simulink model "InnerController"  (R2016b)
settings: Solver=FixedStepAuto  StartTime=0.0  StopTime=t  FixedStep=Ts  RelTol=1e-3
model workspace (MAT data in the model file):
  index = Simulink.Signal
  index.DataType = 'double'
  index.Dimensions = 1
  index.DimensionsMode = 'Fixed'
  index.Complexity = 'real'
  index.SampleTime = -1
  index.SamplingMode = 'auto'
  index.InitialValue = '1'
values from neighbouring files (symbols this model uses):
  dx = 2.86    [Parameters.m]    (also in PlotControllersPerformance.m = dx_rand(i))
  dy = 32.5    [Parameters.m]    (also in PlotControllersPerformance.m = dy_rand(i))
  dyaw = 0.26285    [Parameters.m]    (also in PlotControllersPerformance.m = dyaw_rand(i))
  enable_disturbance = 1    [PlotControllersPerformance.m]
  F_lqr = Fe_lqr(1:2,1:3)    [ControllersDesign.m]
  F_rob = -info.KFI(1:2,1:3)    [ControllersDesign.m]
  FI_lqr = Fe_lqr(1:2,4:5)    [ControllersDesign.m]
  FI_rob = -info.KFI(1:2,4:5)    [ControllersDesign.m]
  Iz = 1.10675    [Parameters.m]    (also in PlotControllersPerformance.m = Iz_rand(i))
  l1 = 0.05    [Parameters.m]    (also in PlotControllersPerformance.m = l1_rand(i))
  l2 = 0.05    [Parameters.m]    (also in PlotControllersPerformance.m = l2_rand(i))
  m = 13    [Parameters.m]    (also in PlotControllersPerformance.m = m_rand(i))
  noise_power_xbdot = 0.000001    (= 1e-06)    [PlotControllersPerformance.m]
  noise_power_yaw = 0.0000001    (= 1e-07)    [PlotControllersPerformance.m]
  noise_power_yawdot = 0.000001    (= 1e-06)    [PlotControllersPerformance.m]
  refXdot = 1    [PlotControllersPerformance.m]
  refYaw = 1    [PlotControllersPerformance.m]
  sineAmplitude = 0.5    [PlotControllersPerformance.m]
  sineFrequency = sineFrequency_rand(i)    [PlotControllersPerformance.m]
  time_step = 10    [PlotControllersPerformance.m]
  Ts = 0.05    [Parameters.m]
  xbDisturbance = xbDisturbance_rand(i)    [PlotControllersPerformance.m]
  yawDisturbance = yawDisturbance_rand(i)    [PlotControllersPerformance.m]
undefined symbols (not defined in the file or in its folder): DiscIntNeverNeededParam
libraries: simulink x6
settings Model: Creator=USUARIO  LastModifiedBy=USUARIO
settings DataIOCC: Refine=100

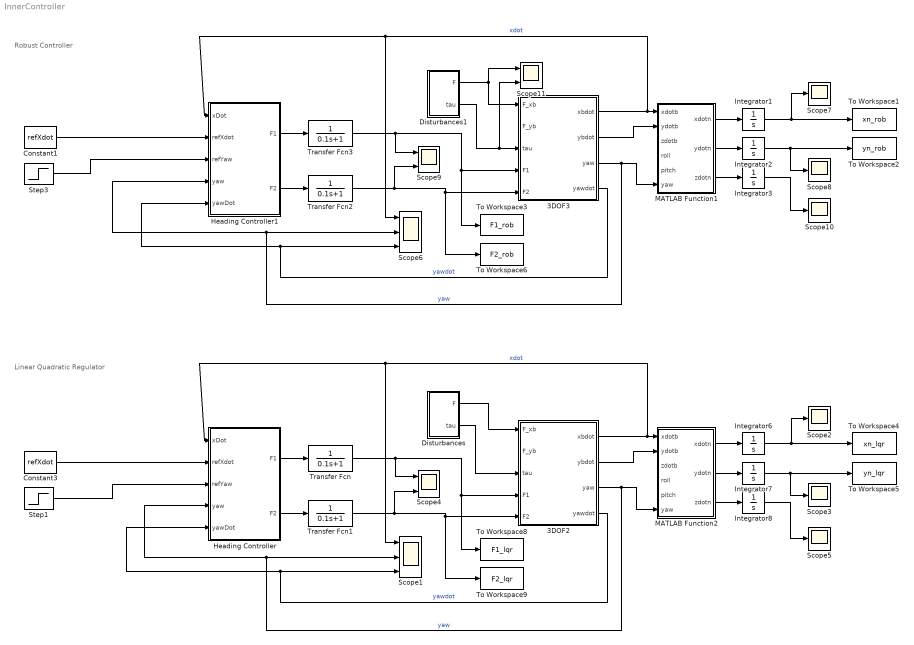
== system InnerController ==
  note: Linear Quadratic Regulator
  note: Robust Controller
  3DOF2 : Subsystem
  3DOF3 : Subsystem
  Constant1 : Constant  Value=refXdot
  Constant3 : Constant  Value=refXdot
  Disturbances : Subsystem
  Disturbances1 : Subsystem
  Heading Controller : Subsystem
  Heading Controller1 : Subsystem
  Integrator{1..3,6..8} (6 alike) : Integrator
  MATLAB Function1 : MATLAB Function  TreatAsAtomicUnit=on
  MATLAB Function2 : MATLAB Function  TreatAsAtomicUnit=on
  Scope1 : Scope  NumInputPorts=3
  Scope{2..3,5,7..8,10} (6 alike) : Scope
  Scope11 : Scope  NumInputPorts=2
  Scope4 : Scope  NumInputPorts=2
  Scope6 : Scope  NumInputPorts=3
  Scope9 : Scope  NumInputPorts=2
  Step1 : Step  Time=time_step  After=refYaw  SampleTime=0
  Step3 : Step  Time=time_step  After=refYaw  SampleTime=0
  To Workspace1 : ToWorkspace  VariableName=xn_rob  SaveFormat=Timeseries  SampleTime=-1
  To Workspace2 : ToWorkspace  VariableName=yn_rob  SaveFormat=Timeseries  SampleTime=-1
  To Workspace3 : ToWorkspace  VariableName=F1_rob  SaveFormat=Timeseries  SampleTime=Ts
  To Workspace4 : ToWorkspace  VariableName=xn_lqr  SaveFormat=Timeseries  SampleTime=-1
  To Workspace5 : ToWorkspace  VariableName=yn_lqr  SaveFormat=Timeseries  SampleTime=-1
  To Workspace6 : ToWorkspace  VariableName=F2_rob  SaveFormat=Timeseries  SampleTime=Ts
  To Workspace8 : ToWorkspace  VariableName=F1_lqr  SaveFormat=Timeseries  SampleTime=-1
  To Workspace9 : ToWorkspace  VariableName=F2_lqr  SaveFormat=Timeseries  SampleTime=-1
  Transfer Fcn{,1..3} (4 alike) : TransferFcn  Denominator=[0.1 1]
  wires:
  3DOF2/1(xbdot) -> Scope1/1, Heading Controller/1(xDot), MATLAB Function2/1(xdotb)  "xdot"
  3DOF2/2(ybdot) -> MATLAB Function2/2(ydotb)
  3DOF2/3(yaw) -> MATLAB Function2/6(yaw), Scope1/2, Heading Controller/4(yaw)  "yaw"
  Integrator6/1 -> Scope2/1, To Workspace4/1
  Integrator7/1 -> Scope3/1, To Workspace5/1
  MATLAB Function2/3(zdotn) -> Integrator8/1
  3DOF2/4(yawdot) -> Heading Controller/5(yawDot), Scope1/3  "yawdot"
  Heading Controller/2(F2) -> Transfer Fcn1/1
  Heading Controller/1(F1) -> Transfer Fcn/1
  MATLAB Function2/1(xdotn) -> Integrator6/1
  MATLAB Function2/2(ydotn) -> Integrator7/1
  Integrator8/1 -> Scope5/1
  Constant3/1 -> Heading Controller/2(refXdot)
  Step1/1 -> Heading Controller/3(refYaw)
  3DOF3/1(xbdot) -> MATLAB Function1/1(xdotb), Scope6/1, Heading Controller1/1(xDot)  "xdot"
  3DOF3/2(ybdot) -> MATLAB Function1/2(ydotb)
  3DOF3/3(yaw) -> Scope6/2, Heading Controller1/4(yaw), MATLAB Function1/6(yaw)  "yaw"
  Integrator1/1 -> To Workspace1/1, Scope7/1
  Integrator2/1 -> To Workspace2/1, Scope8/1
  MATLAB Function1/3(zdotn) -> Integrator3/1
  3DOF3/4(yawdot) -> Scope6/3, Heading Controller1/5(yawDot)  "yawdot"
  Heading Controller1/2(F2) -> Transfer Fcn2/1
  Heading Controller1/1(F1) -> Transfer Fcn3/1
  MATLAB Function1/1(xdotn) -> Integrator1/1
  MATLAB Function1/2(ydotn) -> Integrator2/1
  Integrator3/1 -> Scope10/1
  Constant1/1 -> Heading Controller1/2(refXdot)
  Step3/1 -> Heading Controller1/3(refYaw)
  Transfer Fcn/1 -> Scope4/1, 3DOF2/4(F1), To Workspace8/1
  Transfer Fcn1/1 -> Scope4/2, 3DOF2/5(F2), To Workspace9/1
  Transfer Fcn2/1 -> 3DOF3/5(F2), To Workspace6/1, Scope9/2
  Transfer Fcn3/1 -> 3DOF3/4(F1), To Workspace3/1, Scope9/1
  Disturbances1/1(F) -> 3DOF3/1(F_xb), Scope11/1
  Disturbances1/2(tau) -> Scope11/2, 3DOF3/3(tau)
  Disturbances/1(F) -> 3DOF2/1(F_xb)
  Disturbances/2(tau) -> 3DOF2/3(tau)

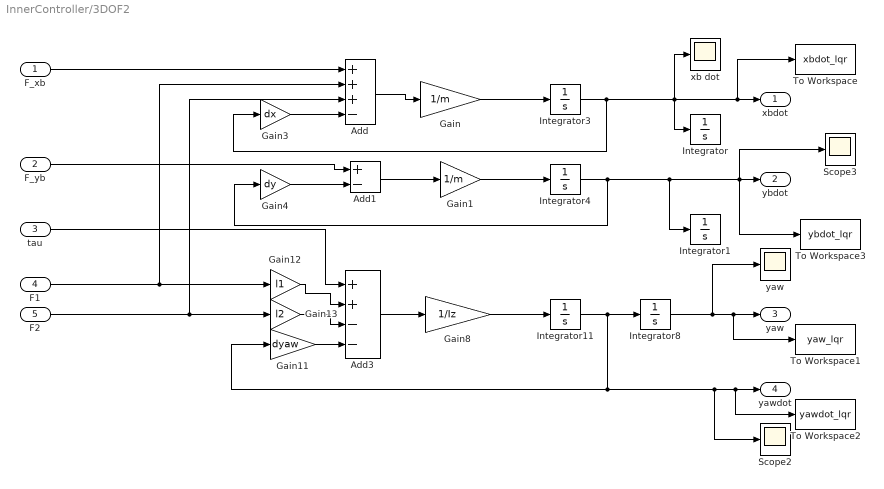
== system InnerController/3DOF2 ==
  F_xb : Inport
  F_yb : Inport  Port=2
  tau : Inport  Port=3
  F1 : Inport  Port=4
  F2 : Inport  Port=5
  Add : Sum  Inputs=+++-
  Add1 : Sum  Inputs=+-
  Add3 : Sum  Inputs=++--
  Gain : Gain  Gain=1/m
  Gain1 : Gain  Gain=1/m
  Gain11 : Gain  Gain=dyaw
  Gain12 : Gain  Gain=l1
  Gain13 : Gain  Gain=l2
  Gain3 : Gain  Gain=dx
  Gain4 : Gain  Gain=dy
  Gain8 : Gain  Gain=1/Iz
  Integrator{,1,3..4,8,11} (6 alike) : Integrator
  Scope2 : Scope
  Scope3 : Scope
  To Workspace : ToWorkspace  VariableName=xbdot_lqr  SaveFormat=Timeseries  SampleTime=Ts
  To Workspace1 : ToWorkspace  VariableName=yaw_lqr  SaveFormat=Timeseries  SampleTime=Ts
  To Workspace2 : ToWorkspace  VariableName=yawdot_lqr  SaveFormat=Timeseries  SampleTime=Ts
  To Workspace3 : ToWorkspace  VariableName=ybdot_lqr  SaveFormat=Timeseries  SampleTime=Ts
  xb dot : Scope
  "yaw " : Scope
  xbdot : Outport
  ybdot : Outport  Port=2
  yaw : Outport  Port=3
  yawdot : Outport  Port=4
  wires:
  Integrator11/1 -> Scope2/1, To Workspace2/1, yawdot/1, Gain11/1, Integrator8/1
  Gain8/1 -> Integrator11/1
  Gain4/1 -> Add1/2
  Gain1/1 -> Integrator4/1
  Gain3/1 -> Add/4
  Add/1 -> Gain/1
  Gain/1 -> Integrator3/1
  Gain12/1 -> Add3/2
  Add3/1 -> Gain8/1
  Gain11/1 -> Add3/4
  Gain13/1 -> Add3/3
  Integrator3/1 -> xb dot/1, Integrator/1, To Workspace/1, xbdot/1, Gain3/1
  Integrator4/1 -> Gain4/1, Integrator1/1, To Workspace3/1, ybdot/1, Scope3/1
  Integrator8/1 -> "yaw "/1, To Workspace1/1, yaw/1
  F1/1 -> Add/2, Gain12/1
  F2/1 -> Add/3, Gain13/1
  Add1/1 -> Gain1/1
  F_yb/1 -> Add1/1
  F_xb/1 -> Add/1
  tau/1 -> Add3/1

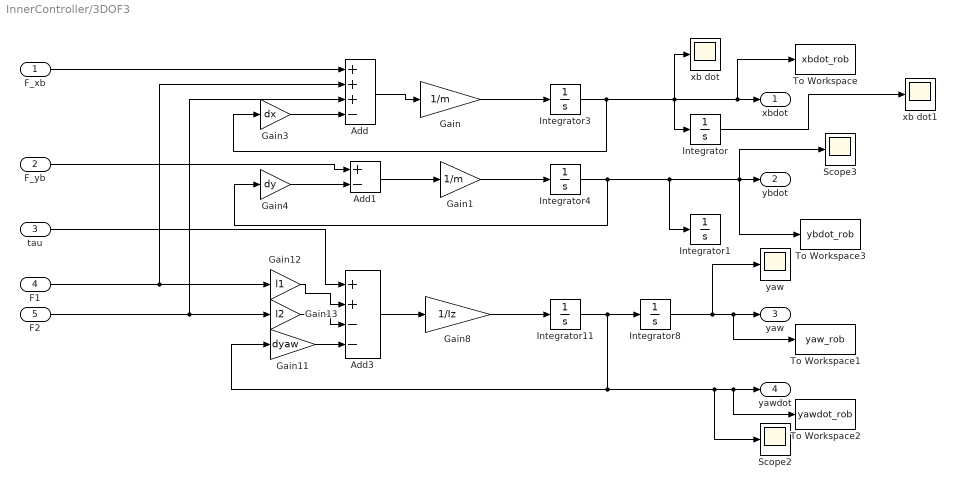
== system InnerController/3DOF3 ==
  F_xb : Inport
  F_yb : Inport  Port=2
  tau : Inport  Port=3
  F1 : Inport  Port=4
  F2 : Inport  Port=5
  Add : Sum  Inputs=+++-
  Add1 : Sum  Inputs=+-
  Add3 : Sum  Inputs=++--
  Gain : Gain  Gain=1/m
  Gain1 : Gain  Gain=1/m
  Gain11 : Gain  Gain=dyaw
  Gain12 : Gain  Gain=l1
  Gain13 : Gain  Gain=l2
  Gain3 : Gain  Gain=dx
  Gain4 : Gain  Gain=dy
  Gain8 : Gain  Gain=1/Iz
  Integrator{,1,3..4,8,11} (6 alike) : Integrator
  Scope2 : Scope
  Scope3 : Scope
  To Workspace : ToWorkspace  VariableName=xbdot_rob  SaveFormat=Timeseries  SampleTime=Ts
  To Workspace1 : ToWorkspace  VariableName=yaw_rob  SaveFormat=Timeseries  SampleTime=Ts
  To Workspace2 : ToWorkspace  VariableName=yawdot_rob  SaveFormat=Timeseries  SampleTime=Ts
  To Workspace3 : ToWorkspace  VariableName=ybdot_rob  SaveFormat=Timeseries  SampleTime=Ts
  xb dot : Scope
  xb dot1 : Scope
  "yaw " : Scope
  xbdot : Outport
  ybdot : Outport  Port=2
  yaw : Outport  Port=3
  yawdot : Outport  Port=4
  wires:
  tau/1 -> Add3/1
  F_xb/1 -> Add/1
  F_yb/1 -> Add1/1
  Add1/1 -> Gain1/1
  F2/1 -> Gain13/1, Add/3
  F1/1 -> Gain12/1, Add/2
  Integrator8/1 -> yaw/1, To Workspace1/1, "yaw "/1
  Integrator4/1 -> Scope3/1, ybdot/1, To Workspace3/1, Integrator1/1, Gain4/1
  Integrator3/1 -> Gain3/1, xbdot/1, To Workspace/1, Integrator/1, xb dot/1
  Gain13/1 -> Add3/3
  Gain11/1 -> Add3/4
  Add3/1 -> Gain8/1
  Gain12/1 -> Add3/2
  Gain/1 -> Integrator3/1
  Add/1 -> Gain/1
  Gain3/1 -> Add/4
  Gain1/1 -> Integrator4/1
  Gain4/1 -> Add1/2
  Gain8/1 -> Integrator11/1
  Integrator11/1 -> Integrator8/1, Gain11/1, To Workspace2/1, yawdot/1, Scope2/1
  Integrator/1 -> xb dot1/1

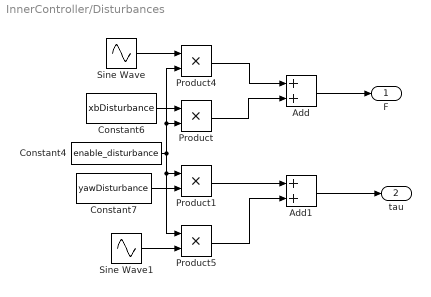
== system InnerController/Disturbances ==
  Add : Sum
  Add1 : Sum
  Constant4 : Constant  Value=enable_disturbance
  Constant6 : Constant  Value=xbDisturbance
  Constant7 : Constant  Value=yawDisturbance
  Product{,1,4..5} (4 alike) : Product
  Sine Wave : Sin  Amplitude=sineAmplitude  Frequency=sineFrequency  SampleTime=0
  Sine Wave1 : Sin  Amplitude=sineAmplitude  Frequency=sineFrequency  SampleTime=0
  F : Outport
  tau : Outport  Port=2
  wires:
  Constant4/1 -> Product5/1, Product1/1, Product4/2, Product/2
  Constant7/1 -> Product1/2
  Product/1 -> Add/2
  Constant6/1 -> Product/1
  Sine Wave/1 -> Product4/1
  Sine Wave1/1 -> Product5/2
  Product5/1 -> Add1/2
  Add/1 -> F/1
  Add1/1 -> tau/1
  Product1/1 -> Add1/1
  Product4/1 -> Add/1

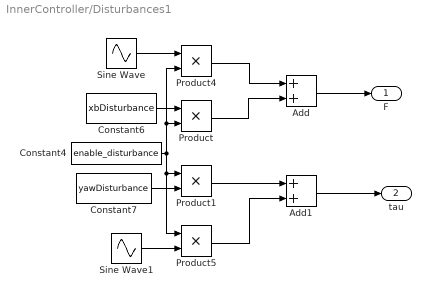
== system InnerController/Disturbances1 ==
  Add : Sum
  Add1 : Sum
  Constant4 : Constant  Value=enable_disturbance
  Constant6 : Constant  Value=xbDisturbance
  Constant7 : Constant  Value=yawDisturbance
  Product{,1,4..5} (4 alike) : Product
  Sine Wave : Sin  Amplitude=sineAmplitude  Frequency=sineFrequency  SampleTime=0
  Sine Wave1 : Sin  Amplitude=sineAmplitude  Frequency=sineFrequency  SampleTime=0
  F : Outport
  tau : Outport  Port=2
  wires:
  Product4/1 -> Add/1
  Product1/1 -> Add1/1
  Add1/1 -> tau/1
  Add/1 -> F/1
  Product5/1 -> Add1/2
  Sine Wave1/1 -> Product5/2
  Sine Wave/1 -> Product4/1
  Constant6/1 -> Product/1
  Product/1 -> Add/2
  Constant7/1 -> Product1/2
  Constant4/1 -> Product/2, Product4/2, Product1/1, Product5/1

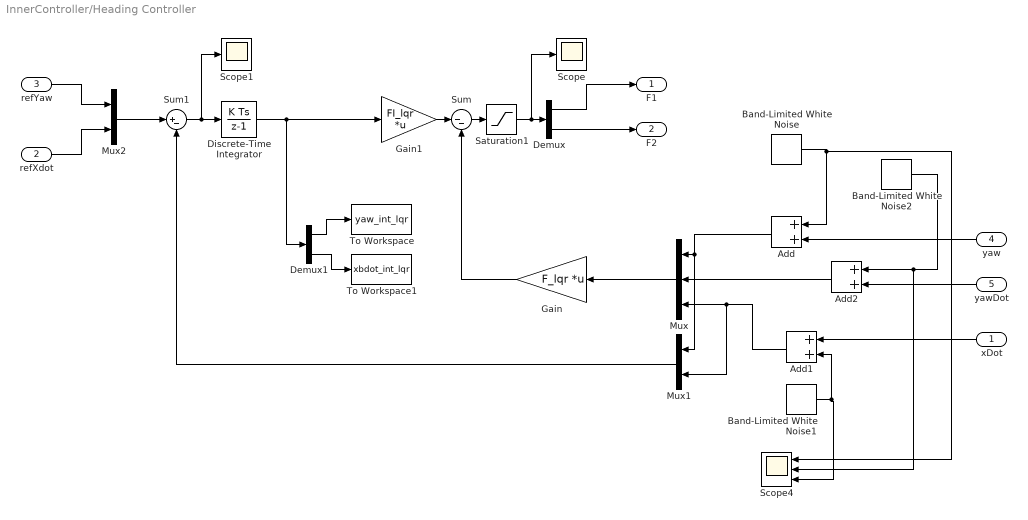
== system InnerController/Heading Controller ==
  xDot : Inport
  refXdot : Inport  Port=2  PortDimensions=1
  refYaw : Inport  Port=3  PortDimensions=1
  yaw : Inport  Port=4
  yawDot : Inport  Port=5
  Add : Sum
  Add1 : Sum
  Add2 : Sum
  Band-Limited White Noise : simulink/Sources/Band-Limited White Noise  Cov=[noise_power_yaw]  Ts=Ts  seed=[23341]
  Band-Limited White Noise1 : simulink/Sources/Band-Limited White Noise  Cov=[noise_power_xbdot]  Ts=Ts  seed=[23041]
  Band-Limited White Noise2 : simulink/Sources/Band-Limited White Noise  Cov=[noise_power_yawdot]  Ts=Ts  seed=[23026]
  Demux : Demux  Outputs=2
  Demux1 : Demux  Outputs=2
  Discrete-Time Integrator : DiscreteIntegrator  InitialConditionSetting=State (most efficient)  SampleTime=-1  ICPrevOutput=DiscIntNeverNeededParam  ICPrevScaledInput=DiscIntNeverNeededParam
  Gain : Gain  Gain=F_lqr  Multiplication=Matrix(K*u)
  Gain1 : Gain  Gain=FI_lqr  Multiplication=Matrix(K*u)
  Mux : Mux  Inputs=3
  Mux1 : Mux  Inputs=2
  Mux2 : Mux  Inputs=2
  Saturation1 : Saturate  UpperLimit=50  LowerLimit=-25
  Scope : Scope
  Scope1 : Scope
  Scope4 : Scope  NumInputPorts=3
  Sum : Sum  Inputs=|--
  Sum1 : Sum  Inputs=|+-
  To Workspace : ToWorkspace  VariableName=yaw_int_lqr  SaveFormat=Timeseries  SampleTime=-1
  To Workspace1 : ToWorkspace  VariableName=xbdot_int_lqr  SaveFormat=Timeseries  SampleTime=-1
  F1 : Outport
  F2 : Outport  Port=2
  wires:
  Saturation1/1 -> Scope/1, Demux/1
  Sum1/1 -> Scope1/1, Discrete-Time Integrator/1
  Demux/1 -> F1/1
  Demux/2 -> F2/1
  Sum/1 -> Saturation1/1
  Gain/1 -> Sum/2
  Mux/1 -> Gain/1
  refYaw/1 -> Mux2/1
  Mux2/1 -> Sum1/1
  Mux1/1 -> Sum1/2
  refXdot/1 -> Mux2/2
  Gain1/1 -> Sum/1
  Discrete-Time Integrator/1 -> Demux1/1, Gain1/1
  Demux1/1 -> To Workspace/1
  Demux1/2 -> To Workspace1/1
  Add1/1 -> Mux/3, Mux1/2
  Band-Limited White Noise1/1 -> Scope4/3, Add1/2
  xDot/1 -> Add1/1
  Band-Limited White Noise/1 -> Scope4/1, Add/1
  yaw/1 -> Add/2
  yawDot/1 -> Add2/2
  Add/1 -> Mux/1, Mux1/1
  Add2/1 -> Mux/2
  Band-Limited White Noise2/1 -> Scope4/2, Add2/1

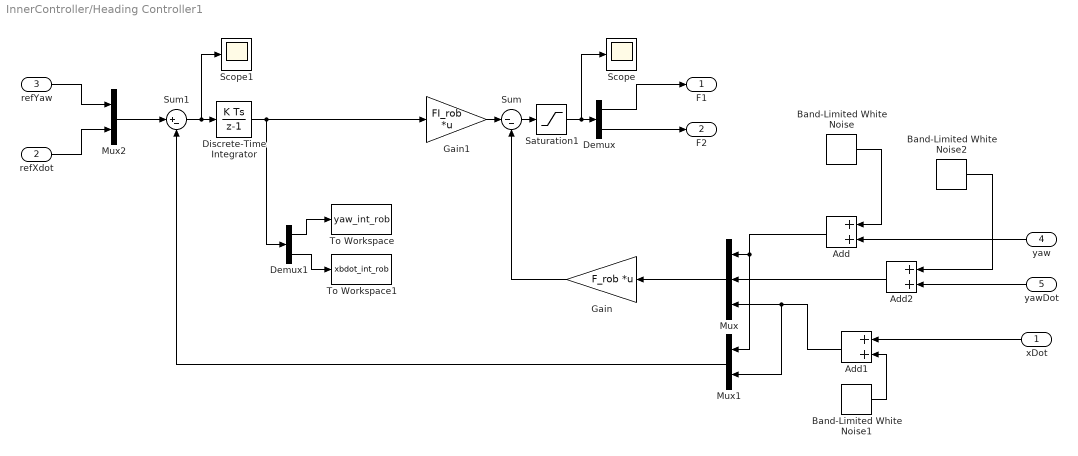
== system InnerController/Heading Controller1 ==
  xDot : Inport
  refXdot : Inport  Port=2  PortDimensions=1
  refYaw : Inport  Port=3  PortDimensions=1
  yaw : Inport  Port=4
  yawDot : Inport  Port=5
  Add : Sum
  Add1 : Sum
  Add2 : Sum
  Band-Limited White Noise : simulink/Sources/Band-Limited White Noise  Cov=[noise_power_yaw]  Ts=Ts  seed=[23341]
  Band-Limited White Noise1 : simulink/Sources/Band-Limited White Noise  Cov=[noise_power_xbdot]  Ts=Ts  seed=[23041]
  Band-Limited White Noise2 : simulink/Sources/Band-Limited White Noise  Cov=[noise_power_yawdot]  Ts=Ts  seed=[23026]
  Demux : Demux  Outputs=2
  Demux1 : Demux  Outputs=2
  Discrete-Time Integrator : DiscreteIntegrator  InitialConditionSetting=State (most efficient)  SampleTime=-1  ICPrevOutput=DiscIntNeverNeededParam  ICPrevScaledInput=DiscIntNeverNeededParam
  Gain : Gain  Gain=F_rob  Multiplication=Matrix(K*u)
  Gain1 : Gain  Gain=FI_rob  Multiplication=Matrix(K*u)
  Mux : Mux  Inputs=3
  Mux1 : Mux  Inputs=2
  Mux2 : Mux  Inputs=2
  Saturation1 : Saturate  UpperLimit=50  LowerLimit=-25
  Scope : Scope
  Scope1 : Scope
  Sum : Sum  Inputs=|--
  Sum1 : Sum  Inputs=|+-
  To Workspace : ToWorkspace  VariableName=yaw_int_rob  SaveFormat=Timeseries  SampleTime=-1
  To Workspace1 : ToWorkspace  VariableName=xbdot_int_rob  SaveFormat=Timeseries  SampleTime=-1
  F1 : Outport
  F2 : Outport  Port=2
  wires:
  Gain1/1 -> Sum/1
  Add1/1 -> Mux1/2, Mux/3
  Band-Limited White Noise1/1 -> Add1/2
  xDot/1 -> Add1/1
  Band-Limited White Noise/1 -> Add/1
  yaw/1 -> Add/2
  refXdot/1 -> Mux2/2
  Mux1/1 -> Sum1/2
  Mux2/1 -> Sum1/1
  refYaw/1 -> Mux2/1
  Mux/1 -> Gain/1
  Gain/1 -> Sum/2
  Sum/1 -> Saturation1/1
  yawDot/1 -> Add2/2
  Discrete-Time Integrator/1 -> Demux1/1, Gain1/1
  Demux/2 -> F2/1
  Demux/1 -> F1/1
  Sum1/1 -> Scope1/1, Discrete-Time Integrator/1
  Add/1 -> Mux/1, Mux1/1
  Saturation1/1 -> Demux/1, Scope/1
  Demux1/1 -> To Workspace/1
  Demux1/2 -> To Workspace1/1
  Add2/1 -> Mux/2
  Band-Limited White Noise2/1 -> Add2/1

== matlab function InnerController/MATLAB Function1 ==
  data: xdotb input; xdotn output; ydotb input; zdotb input; roll input; pitch input; yaw input; ydotn output; zdotn output
function [xdotn,ydotn,zdotn] = fcn(xdotb,ydotb,zdotb,roll,pitch,yaw)
R=[cos(pitch)*cos(yaw) sin(roll)*sin(pitch)*cos(yaw)-cos(roll)*sin(yaw) ...
                          cos(roll)*sin(pitch)*cos(yaw)+sin(roll)*sin(yaw);
   cos(pitch)*sin(yaw) sin(roll)*sin(pitch)*sin(yaw)+cos(roll)*cos(yaw) ...
                          cos(roll)*sin(pitch)*sin(yaw)-sin(roll)*cos(yaw);
   -sin(pitch) sin(roll)*cos(pitch) cos(roll)*cos(pitch)];

n=R*[xdotb;ydotb;zdotb];

xdotn=n(1);
ydotn=n(2);
zdotn=n(3);
end

== matlab function InnerController/MATLAB Function2 ==
  data: xdotb input; xdotn output; ydotb input; zdotb input; roll input; pitch input; yaw input; ydotn output; zdotn output
function [xdotn,ydotn,zdotn] = fcn(xdotb,ydotb,zdotb,roll,pitch,yaw)
R=[cos(pitch)*cos(yaw) sin(roll)*sin(pitch)*cos(yaw)-cos(roll)*sin(yaw) ...
                          cos(roll)*sin(pitch)*cos(yaw)+sin(roll)*sin(yaw);
   cos(pitch)*sin(yaw) sin(roll)*sin(pitch)*sin(yaw)+cos(roll)*cos(yaw) ...
                          cos(roll)*sin(pitch)*sin(yaw)-sin(roll)*cos(yaw);
   -sin(pitch) sin(roll)*cos(pitch) cos(roll)*cos(pitch)];

n=R*[xdotb;ydotb;zdotb];

xdotn=n(1);
ydotn=n(2);
zdotn=n(3);
end
